simulink model "t04_combine_gaits_sol"  (R2024b)
settings: Solver=ode23t  StartTime=0.0  StopTime=4  RelTol=1e-3  AbsTol=1e-3  EnableMultiTasking=on
model workspace (MAT data in the model file):
  A = 0.4
  Critical_Velocity = 0.01
  Damping_Factor = 1000
  Dynamic_Friction = 0.5
  Heigth_brick : Simulink.Parameter (value not decoded)
  Heigth_ramp : Simulink.Parameter (value not decoded)
  Length_brick : Simulink.Parameter (value not decoded)
  Length_ramp : Simulink.Parameter (value not decoded)
  Length_torso : Simulink.Parameter (value not decoded)
  Lower_limbs : Simulink.Parameter (value not decoded)
  Static_Friction = 0.7
  Stiffnesscoefficient = 10000
  Transition_Region_Width = 0.02
  Upper_limbs : Simulink.Parameter (value not decoded)
  Width_brick : Simulink.Parameter (value not decoded)
  Width_ramp : Simulink.Parameter (value not decoded)
  Width_torso : Simulink.Parameter (value not decoded)
  f = 1.5
  max_Joint_change = 100
  r_foot : Simulink.Parameter (value not decoded)
  sampleTime : Simulink.Parameter (value not decoded)
  t_leg : Simulink.Parameter (value not decoded)
  theta : Simulink.Parameter (value not decoded)
  transferFunVal : Simulink.Parameter (value not decoded)
symbols that are objects in the model workspace (value not decoded): Length_torso, Lower_limbs, t_leg, Upper_limbs, Width_torso
undefined symbols (not defined in the file): X, Y, Z
libraries: sm_lib x78, nesl_utility x13
(part 3 of 4)

== system t04_combine_gaits_sol/Front left leg/Upper Limb ==
  BaseUpperLimb : sm_lib/Body Elements/Brick Solid  BrickDimensions=[t_leg t_leg L]  BrickDimensionsUnits=m  ExportEntireGeometry=off  InertiaType=CalculateFromGeometry  BasedOnType=Density  Density=1000  DensityUnits=kg/m^3  Mass=1  MassUnits=kg  CenterOfMass=[0 0 0]  CenterOfMassUnits=m  MomentsOfInertia=[1 1 1]  MomentsOfInertiaUnits=kg*m^2  ProductsOfInertia=[0 0 0]  ProductsOfInertiaUnits=kg*m^2  GraphicType=FromGeometry  MarkerShape=Sphere  MarkerSize=10  GraphicVisPropType=SimpleVisualProperties  GraphicDiffuseColor=[0.3922 0.8314 0.07451]  GraphicOpacity=1  GraphicSpecularColor=[0.5 0.5 0.5 1.0]  GraphicAmbientColor=[0.15 0.15 0.15 1.0]  GraphicEmissiveColor=[0.0 0.0 0.0 1.0]  GraphicShininess=75  DoExposeReferenceFrame=off  SerializedFrames=<Frames><Frame><Id>Frame1</Id><Value><Name>B</Name><Origin><Source>GeometricFeature</Source><FeatureName>+z surface</FeatureName></Origin><PrimaryAxis><DefinedDirection>+Z</DefinedDirection><Source>ReferenceFrame</Source><SourceDirection>+Z</SourceDirection><FeatureName></FeatureName></PrimaryAxis><SecondaryAxis><DefinedDirection>+X</DefinedDirection><Source>ReferenceFrame</Source><SourceDirection>+X</SourceDirection><FeatureName></FeatureName></SecondaryAxis></Value></Frame><Frame><Id>Frame2</Id><Value><Name>F</Name><Origin><Source>GeometricFeature</Source><FeatureName>-z surface</FeatureName></Origin><PrimaryAxis><DefinedDirection>+Z</DefinedDirection><Source>ReferenceFrame</Source><SourceDirection>+Z</SourceDirection><FeatureName></FeatureName></PrimaryAxis><SecondaryAxis><DefinedDirection>+X</DefinedDirection><Source>ReferenceFrame</Source><SourceDirection>+X</SourceDirection><FeatureName></FeatureName></SecondaryAxis></Value></Frame></Frames>
  Transform Shoulder : sm_lib/Frames and Transforms/Rigid Transform  RotationMethod=StandardAxis  FollAlignAxisA=+X  BaseAlignAxisA=+Y  FollAlignAxisB=+Y  BaseAlignAxisB=+Z  RotationStandardAxis=+X  RotationAngle=-90  RotationAngleUnits=deg  RotationArbitraryAxis=[0 0 1]  RotationSequenceAxes=FollowerAxes  RotationSequence=XYX  RotationSequenceAngles=[0 0 0]  RotationSequenceAnglesUnits=deg  RotationMatrix=[1 0 0;0 1 0;0 0 1]  Quaternion=[1 0 0 0]  TranslationMethod=StandardAxis  TranslationCartesianOffset=[0 0 0]  TranslationCartesianOffsetUnits=m  TranslationStandardAxis=+Z  TranslationStandardOffset=0  TranslationStandardOffsetUnits=m  TranslationROffset=0  TranslationROffsetUnits=m  TranslationThetaOffset=0  TranslationThetaOffsetUnits=deg  TranslationZOffset=0  TranslationZOffsetUnits=m
  Transform Upper Knee : sm_lib/Frames and Transforms/Rigid Transform  RotationMethod=StandardAxis  FollAlignAxisA=+X  BaseAlignAxisA=+Y  FollAlignAxisB=+Y  BaseAlignAxisB=+Z  RotationStandardAxis=+X  RotationAngle=-90  RotationAngleUnits=deg  RotationArbitraryAxis=[0 0 1]  RotationSequenceAxes=FollowerAxes  RotationSequence=XYX  RotationSequenceAngles=[0 0 0]  RotationSequenceAnglesUnits=deg  RotationMatrix=[1 0 0;0 1 0;0 0 1]  Quaternion=[1 0 0 0]  TranslationMethod=StandardAxis  TranslationCartesianOffset=[0 0 0]  TranslationCartesianOffsetUnits=m  TranslationStandardAxis=+Z  TranslationStandardOffset=0  TranslationStandardOffsetUnits=m  TranslationROffset=0  TranslationROffsetUnits=m  TranslationThetaOffset=0  TranslationThetaOffsetUnits=deg  TranslationZOffset=0  TranslationZOffsetUnits=m
  U : PMIOPort  Side=Left
  L : PMIOPort  Port=2  Side=Right
  connections:
  L/RConn1 -- Transform Upper Knee/RConn1
  U/RConn1 -- Transform Shoulder/RConn1
  BaseUpperLimb/LConn1 -- Transform Shoulder/LConn1
  BaseUpperLimb/RConn1 -- Transform Upper Knee/LConn1

== system t04_combine_gaits_sol/Front right leg/Lower Limb ==
  BaseLowerLimb : sm_lib/Body Elements/Brick Solid  BrickDimensions=[t_leg t_leg L]  BrickDimensionsUnits=m  ExportEntireGeometry=off  InertiaType=CalculateFromGeometry  BasedOnType=Density  Density=1000  DensityUnits=kg/m^3  Mass=1  MassUnits=kg  CenterOfMass=[0 0 0]  CenterOfMassUnits=m  MomentsOfInertia=[1 1 1]  MomentsOfInertiaUnits=kg*m^2  ProductsOfInertia=[0 0 0]  ProductsOfInertiaUnits=kg*m^2  GraphicType=FromGeometry  MarkerShape=Sphere  MarkerSize=10  GraphicVisPropType=SimpleVisualProperties  GraphicDiffuseColor=[0.3922 0.8314 0.07451]  GraphicOpacity=1  GraphicSpecularColor=[0.5 0.5 0.5 1.0]  GraphicAmbientColor=[0.15 0.15 0.15 1.0]  GraphicEmissiveColor=[0.0 0.0 0.0 1.0]  GraphicShininess=75  DoExposeReferenceFrame=off  SerializedFrames=<Frames><Frame><Id>Frame1</Id><Value><Name>B</Name><Origin><Source>GeometricFeature</Source><FeatureName>+z surface</FeatureName></Origin><PrimaryAxis><DefinedDirection>+Z</DefinedDirection><Source>ReferenceFrame</Source><SourceDirection>+Z</SourceDirection><FeatureName></FeatureName></PrimaryAxis><SecondaryAxis><DefinedDirection>+X</DefinedDirection><Source>ReferenceFrame</Source><SourceDirection>+X</SourceDirection><FeatureName></FeatureName></SecondaryAxis></Value></Frame><Frame><Id>Frame2</Id><Value><Name>F</Name><Origin><Source>GeometricFeature</Source><FeatureName>-z surface</FeatureName></Origin><PrimaryAxis><DefinedDirection>+Z</DefinedDirection><Source>ReferenceFrame</Source><SourceDirection>+Z</SourceDirection><FeatureName></FeatureName></PrimaryAxis><SecondaryAxis><DefinedDirection>+X</DefinedDirection><Source>ReferenceFrame</Source><SourceDirection>+X</SourceDirection><FeatureName></FeatureName></SecondaryAxis></Value></Frame></Frames>
  Transform Shoulder : sm_lib/Frames and Transforms/Rigid Transform  RotationMethod=StandardAxis  FollAlignAxisA=+X  BaseAlignAxisA=+Y  FollAlignAxisB=+Y  BaseAlignAxisB=+Z  RotationStandardAxis=+X  RotationAngle=-90  RotationAngleUnits=deg  RotationArbitraryAxis=[0 0 1]  RotationSequenceAxes=FollowerAxes  RotationSequence=XYX  RotationSequenceAngles=[0 0 0]  RotationSequenceAnglesUnits=deg  RotationMatrix=[1 0 0;0 1 0;0 0 1]  Quaternion=[1 0 0 0]  TranslationMethod=StandardAxis  TranslationCartesianOffset=[0 0 0]  TranslationCartesianOffsetUnits=m  TranslationStandardAxis=+Z  TranslationStandardOffset=0  TranslationStandardOffsetUnits=m  TranslationROffset=0  TranslationROffsetUnits=m  TranslationThetaOffset=0  TranslationThetaOffsetUnits=deg  TranslationZOffset=0  TranslationZOffsetUnits=m
  Transform Upper Knee : sm_lib/Frames and Transforms/Rigid Transform  RotationMethod=StandardAxis  FollAlignAxisA=+X  BaseAlignAxisA=+Y  FollAlignAxisB=+Y  BaseAlignAxisB=+Z  RotationStandardAxis=+X  RotationAngle=-90  RotationAngleUnits=deg  RotationArbitraryAxis=[0 0 1]  RotationSequenceAxes=FollowerAxes  RotationSequence=XYX  RotationSequenceAngles=[0 0 0]  RotationSequenceAnglesUnits=deg  RotationMatrix=[1 0 0;0 1 0;0 0 1]  Quaternion=[1 0 0 0]  TranslationMethod=StandardAxis  TranslationCartesianOffset=[0 0 0]  TranslationCartesianOffsetUnits=m  TranslationStandardAxis=+Z  TranslationStandardOffset=0  TranslationStandardOffsetUnits=m  TranslationROffset=0  TranslationROffsetUnits=m  TranslationThetaOffset=0  TranslationThetaOffsetUnits=deg  TranslationZOffset=0  TranslationZOffsetUnits=m
  U : PMIOPort  Side=Left
  L : PMIOPort  Port=2  Side=Right
  connections:
  BaseLowerLimb/LConn1 -- Transform Shoulder/LConn1
  Transform Shoulder/RConn1 -- U/RConn1
  L/RConn1 -- Transform Upper Knee/RConn1
  BaseLowerLimb/RConn1 -- Transform Upper Knee/LConn1

== system t04_combine_gaits_sol/Front right leg/Upper Limb ==
  BaseUpperLimb : sm_lib/Body Elements/Brick Solid  BrickDimensions=[t_leg t_leg L]  BrickDimensionsUnits=m  ExportEntireGeometry=off  InertiaType=CalculateFromGeometry  BasedOnType=Density  Density=1000  DensityUnits=kg/m^3  Mass=1  MassUnits=kg  CenterOfMass=[0 0 0]  CenterOfMassUnits=m  MomentsOfInertia=[1 1 1]  MomentsOfInertiaUnits=kg*m^2  ProductsOfInertia=[0 0 0]  ProductsOfInertiaUnits=kg*m^2  GraphicType=FromGeometry  MarkerShape=Sphere  MarkerSize=10  GraphicVisPropType=SimpleVisualProperties  GraphicDiffuseColor=[0.3922 0.8314 0.07451]  GraphicOpacity=1  GraphicSpecularColor=[0.5 0.5 0.5 1.0]  GraphicAmbientColor=[0.15 0.15 0.15 1.0]  GraphicEmissiveColor=[0.0 0.0 0.0 1.0]  GraphicShininess=75  DoExposeReferenceFrame=off  SerializedFrames=<Frames><Frame><Id>Frame1</Id><Value><Name>B</Name><Origin><Source>GeometricFeature</Source><FeatureName>+z surface</FeatureName></Origin><PrimaryAxis><DefinedDirection>+Z</DefinedDirection><Source>ReferenceFrame</Source><SourceDirection>+Z</SourceDirection><FeatureName></FeatureName></PrimaryAxis><SecondaryAxis><DefinedDirection>+X</DefinedDirection><Source>ReferenceFrame</Source><SourceDirection>+X</SourceDirection><FeatureName></FeatureName></SecondaryAxis></Value></Frame><Frame><Id>Frame2</Id><Value><Name>F</Name><Origin><Source>GeometricFeature</Source><FeatureName>-z surface</FeatureName></Origin><PrimaryAxis><DefinedDirection>+Z</DefinedDirection><Source>ReferenceFrame</Source><SourceDirection>+Z</SourceDirection><FeatureName></FeatureName></PrimaryAxis><SecondaryAxis><DefinedDirection>+X</DefinedDirection><Source>ReferenceFrame</Source><SourceDirection>+X</SourceDirection><FeatureName></FeatureName></SecondaryAxis></Value></Frame></Frames>
  Transform Shoulder : sm_lib/Frames and Transforms/Rigid Transform  RotationMethod=StandardAxis  FollAlignAxisA=+X  BaseAlignAxisA=+Y  FollAlignAxisB=+Y  BaseAlignAxisB=+Z  RotationStandardAxis=+X  RotationAngle=-90  RotationAngleUnits=deg  RotationArbitraryAxis=[0 0 1]  RotationSequenceAxes=FollowerAxes  RotationSequence=XYX  RotationSequenceAngles=[0 0 0]  RotationSequenceAnglesUnits=deg  RotationMatrix=[1 0 0;0 1 0;0 0 1]  Quaternion=[1 0 0 0]  TranslationMethod=StandardAxis  TranslationCartesianOffset=[0 0 0]  TranslationCartesianOffsetUnits=m  TranslationStandardAxis=+Z  TranslationStandardOffset=0  TranslationStandardOffsetUnits=m  TranslationROffset=0  TranslationROffsetUnits=m  TranslationThetaOffset=0  TranslationThetaOffsetUnits=deg  TranslationZOffset=0  TranslationZOffsetUnits=m
  Transform Upper Knee : sm_lib/Frames and Transforms/Rigid Transform  RotationMethod=StandardAxis  FollAlignAxisA=+X  BaseAlignAxisA=+Y  FollAlignAxisB=+Y  BaseAlignAxisB=+Z  RotationStandardAxis=+X  RotationAngle=-90  RotationAngleUnits=deg  RotationArbitraryAxis=[0 0 1]  RotationSequenceAxes=FollowerAxes  RotationSequence=XYX  RotationSequenceAngles=[0 0 0]  RotationSequenceAnglesUnits=deg  RotationMatrix=[1 0 0;0 1 0;0 0 1]  Quaternion=[1 0 0 0]  TranslationMethod=StandardAxis  TranslationCartesianOffset=[0 0 0]  TranslationCartesianOffsetUnits=m  TranslationStandardAxis=+Z  TranslationStandardOffset=0  TranslationStandardOffsetUnits=m  TranslationROffset=0  TranslationROffsetUnits=m  TranslationThetaOffset=0  TranslationThetaOffsetUnits=deg  TranslationZOffset=0  TranslationZOffsetUnits=m
  U : PMIOPort  Side=Left
  L : PMIOPort  Port=2  Side=Right
  connections:
  L/RConn1 -- Transform Upper Knee/RConn1
  U/RConn1 -- Transform Shoulder/RConn1
  BaseUpperLimb/LConn1 -- Transform Shoulder/LConn1
  BaseUpperLimb/RConn1 -- Transform Upper Knee/LConn1

== system t04_combine_gaits_sol/Rear left leg/Lower Limb ==
  BaseLowerLimb : sm_lib/Body Elements/Brick Solid  BrickDimensions=[t_leg t_leg L]  BrickDimensionsUnits=m  ExportEntireGeometry=off  InertiaType=CalculateFromGeometry  BasedOnType=Density  Density=1000  DensityUnits=kg/m^3  Mass=1  MassUnits=kg  CenterOfMass=[0 0 0]  CenterOfMassUnits=m  MomentsOfInertia=[1 1 1]  MomentsOfInertiaUnits=kg*m^2  ProductsOfInertia=[0 0 0]  ProductsOfInertiaUnits=kg*m^2  GraphicType=FromGeometry  MarkerShape=Sphere  MarkerSize=10  GraphicVisPropType=SimpleVisualProperties  GraphicDiffuseColor=[0.3922 0.8314 0.07451]  GraphicOpacity=1  GraphicSpecularColor=[0.5 0.5 0.5 1.0]  GraphicAmbientColor=[0.15 0.15 0.15 1.0]  GraphicEmissiveColor=[0.0 0.0 0.0 1.0]  GraphicShininess=75  DoExposeReferenceFrame=off  SerializedFrames=<Frames><Frame><Id>Frame1</Id><Value><Name>B</Name><Origin><Source>GeometricFeature</Source><FeatureName>+z surface</FeatureName></Origin><PrimaryAxis><DefinedDirection>+Z</DefinedDirection><Source>ReferenceFrame</Source><SourceDirection>+Z</SourceDirection><FeatureName></FeatureName></PrimaryAxis><SecondaryAxis><DefinedDirection>+X</DefinedDirection><Source>ReferenceFrame</Source><SourceDirection>+X</SourceDirection><FeatureName></FeatureName></SecondaryAxis></Value></Frame><Frame><Id>Frame2</Id><Value><Name>F</Name><Origin><Source>GeometricFeature</Source><FeatureName>-z surface</FeatureName></Origin><PrimaryAxis><DefinedDirection>+Z</DefinedDirection><Source>ReferenceFrame</Source><SourceDirection>+Z</SourceDirection><FeatureName></FeatureName></PrimaryAxis><SecondaryAxis><DefinedDirection>+X</DefinedDirection><Source>ReferenceFrame</Source><SourceDirection>+X</SourceDirection><FeatureName></FeatureName></SecondaryAxis></Value></Frame></Frames>
  Transform Shoulder : sm_lib/Frames and Transforms/Rigid Transform  RotationMethod=StandardAxis  FollAlignAxisA=+X  BaseAlignAxisA=+Y  FollAlignAxisB=+Y  BaseAlignAxisB=+Z  RotationStandardAxis=+X  RotationAngle=-90  RotationAngleUnits=deg  RotationArbitraryAxis=[0 0 1]  RotationSequenceAxes=FollowerAxes  RotationSequence=XYX  RotationSequenceAngles=[0 0 0]  RotationSequenceAnglesUnits=deg  RotationMatrix=[1 0 0;0 1 0;0 0 1]  Quaternion=[1 0 0 0]  TranslationMethod=StandardAxis  TranslationCartesianOffset=[0 0 0]  TranslationCartesianOffsetUnits=m  TranslationStandardAxis=+Z  TranslationStandardOffset=0  TranslationStandardOffsetUnits=m  TranslationROffset=0  TranslationROffsetUnits=m  TranslationThetaOffset=0  TranslationThetaOffsetUnits=deg  TranslationZOffset=0  TranslationZOffsetUnits=m
  Transform Upper Knee : sm_lib/Frames and Transforms/Rigid Transform  RotationMethod=StandardAxis  FollAlignAxisA=+X  BaseAlignAxisA=+Y  FollAlignAxisB=+Y  BaseAlignAxisB=+Z  RotationStandardAxis=+X  RotationAngle=-90  RotationAngleUnits=deg  RotationArbitraryAxis=[0 0 1]  RotationSequenceAxes=FollowerAxes  RotationSequence=XYX  RotationSequenceAngles=[0 0 0]  RotationSequenceAnglesUnits=deg  RotationMatrix=[1 0 0;0 1 0;0 0 1]  Quaternion=[1 0 0 0]  TranslationMethod=StandardAxis  TranslationCartesianOffset=[0 0 0]  TranslationCartesianOffsetUnits=m  TranslationStandardAxis=+Z  TranslationStandardOffset=0  TranslationStandardOffsetUnits=m  TranslationROffset=0  TranslationROffsetUnits=m  TranslationThetaOffset=0  TranslationThetaOffsetUnits=deg  TranslationZOffset=0  TranslationZOffsetUnits=m
  U : PMIOPort  Side=Left
  L : PMIOPort  Port=2  Side=Right
  connections:
  BaseLowerLimb/LConn1 -- Transform Shoulder/LConn1
  Transform Shoulder/RConn1 -- U/RConn1
  L/RConn1 -- Transform Upper Knee/RConn1
  BaseLowerLimb/RConn1 -- Transform Upper Knee/LConn1

== system t04_combine_gaits_sol/Rear left leg/Upper Limb ==
  BaseUpperLimb : sm_lib/Body Elements/Brick Solid  BrickDimensions=[t_leg t_leg L]  BrickDimensionsUnits=m  ExportEntireGeometry=off  InertiaType=CalculateFromGeometry  BasedOnType=Density  Density=1000  DensityUnits=kg/m^3  Mass=1  MassUnits=kg  CenterOfMass=[0 0 0]  CenterOfMassUnits=m  MomentsOfInertia=[1 1 1]  MomentsOfInertiaUnits=kg*m^2  ProductsOfInertia=[0 0 0]  ProductsOfInertiaUnits=kg*m^2  GraphicType=FromGeometry  MarkerShape=Sphere  MarkerSize=10  GraphicVisPropType=SimpleVisualProperties  GraphicDiffuseColor=[0.3922 0.8314 0.07451]  GraphicOpacity=1  GraphicSpecularColor=[0.5 0.5 0.5 1.0]  GraphicAmbientColor=[0.15 0.15 0.15 1.0]  GraphicEmissiveColor=[0.0 0.0 0.0 1.0]  GraphicShininess=75  DoExposeReferenceFrame=off  SerializedFrames=<Frames><Frame><Id>Frame1</Id><Value><Name>B</Name><Origin><Source>GeometricFeature</Source><FeatureName>+z surface</FeatureName></Origin><PrimaryAxis><DefinedDirection>+Z</DefinedDirection><Source>ReferenceFrame</Source><SourceDirection>+Z</SourceDirection><FeatureName></FeatureName></PrimaryAxis><SecondaryAxis><DefinedDirection>+X</DefinedDirection><Source>ReferenceFrame</Source><SourceDirection>+X</SourceDirection><FeatureName></FeatureName></SecondaryAxis></Value></Frame><Frame><Id>Frame2</Id><Value><Name>F</Name><Origin><Source>GeometricFeature</Source><FeatureName>-z surface</FeatureName></Origin><PrimaryAxis><DefinedDirection>+Z</DefinedDirection><Source>ReferenceFrame</Source><SourceDirection>+Z</SourceDirection><FeatureName></FeatureName></PrimaryAxis><SecondaryAxis><DefinedDirection>+X</DefinedDirection><Source>ReferenceFrame</Source><SourceDirection>+X</SourceDirection><FeatureName></FeatureName></SecondaryAxis></Value></Frame></Frames>
  Transform Shoulder : sm_lib/Frames and Transforms/Rigid Transform  RotationMethod=StandardAxis  FollAlignAxisA=+X  BaseAlignAxisA=+Y  FollAlignAxisB=+Y  BaseAlignAxisB=+Z  RotationStandardAxis=+X  RotationAngle=-90  RotationAngleUnits=deg  RotationArbitraryAxis=[0 0 1]  RotationSequenceAxes=FollowerAxes  RotationSequence=XYX  RotationSequenceAngles=[0 0 0]  RotationSequenceAnglesUnits=deg  RotationMatrix=[1 0 0;0 1 0;0 0 1]  Quaternion=[1 0 0 0]  TranslationMethod=StandardAxis  TranslationCartesianOffset=[0 0 0]  TranslationCartesianOffsetUnits=m  TranslationStandardAxis=+Z  TranslationStandardOffset=0  TranslationStandardOffsetUnits=m  TranslationROffset=0  TranslationROffsetUnits=m  TranslationThetaOffset=0  TranslationThetaOffsetUnits=deg  TranslationZOffset=0  TranslationZOffsetUnits=m
  Transform Upper Knee : sm_lib/Frames and Transforms/Rigid Transform  RotationMethod=StandardAxis  FollAlignAxisA=+X  BaseAlignAxisA=+Y  FollAlignAxisB=+Y  BaseAlignAxisB=+Z  RotationStandardAxis=+X  RotationAngle=-90  RotationAngleUnits=deg  RotationArbitraryAxis=[0 0 1]  RotationSequenceAxes=FollowerAxes  RotationSequence=XYX  RotationSequenceAngles=[0 0 0]  RotationSequenceAnglesUnits=deg  RotationMatrix=[1 0 0;0 1 0;0 0 1]  Quaternion=[1 0 0 0]  TranslationMethod=StandardAxis  TranslationCartesianOffset=[0 0 0]  TranslationCartesianOffsetUnits=m  TranslationStandardAxis=+Z  TranslationStandardOffset=0  TranslationStandardOffsetUnits=m  TranslationROffset=0  TranslationROffsetUnits=m  TranslationThetaOffset=0  TranslationThetaOffsetUnits=deg  TranslationZOffset=0  TranslationZOffsetUnits=m
  U : PMIOPort  Side=Left
  L : PMIOPort  Port=2  Side=Right
  connections:
  L/RConn1 -- Transform Upper Knee/RConn1
  U/RConn1 -- Transform Shoulder/RConn1
  BaseUpperLimb/LConn1 -- Transform Shoulder/LConn1
  BaseUpperLimb/RConn1 -- Transform Upper Knee/LConn1

== system t04_combine_gaits_sol/Rear right leg/Lower Limb ==
  BaseLowerLimb : sm_lib/Body Elements/Brick Solid  BrickDimensions=[t_leg t_leg L]  BrickDimensionsUnits=m  ExportEntireGeometry=off  InertiaType=CalculateFromGeometry  BasedOnType=Density  Density=1000  DensityUnits=kg/m^3  Mass=1  MassUnits=kg  CenterOfMass=[0 0 0]  CenterOfMassUnits=m  MomentsOfInertia=[1 1 1]  MomentsOfInertiaUnits=kg*m^2  ProductsOfInertia=[0 0 0]  ProductsOfInertiaUnits=kg*m^2  GraphicType=FromGeometry  MarkerShape=Sphere  MarkerSize=10  GraphicVisPropType=SimpleVisualProperties  GraphicDiffuseColor=[0.3922 0.8314 0.07451]  GraphicOpacity=1  GraphicSpecularColor=[0.5 0.5 0.5 1.0]  GraphicAmbientColor=[0.15 0.15 0.15 1.0]  GraphicEmissiveColor=[0.0 0.0 0.0 1.0]  GraphicShininess=75  DoExposeReferenceFrame=off  SerializedFrames=<Frames><Frame><Id>Frame1</Id><Value><Name>B</Name><Origin><Source>GeometricFeature</Source><FeatureName>+z surface</FeatureName></Origin><PrimaryAxis><DefinedDirection>+Z</DefinedDirection><Source>ReferenceFrame</Source><SourceDirection>+Z</SourceDirection><FeatureName></FeatureName></PrimaryAxis><SecondaryAxis><DefinedDirection>+X</DefinedDirection><Source>ReferenceFrame</Source><SourceDirection>+X</SourceDirection><FeatureName></FeatureName></SecondaryAxis></Value></Frame><Frame><Id>Frame2</Id><Value><Name>F</Name><Origin><Source>GeometricFeature</Source><FeatureName>-z surface</FeatureName></Origin><PrimaryAxis><DefinedDirection>+Z</DefinedDirection><Source>ReferenceFrame</Source><SourceDirection>+Z</SourceDirection><FeatureName></FeatureName></PrimaryAxis><SecondaryAxis><DefinedDirection>+X</DefinedDirection><Source>ReferenceFrame</Source><SourceDirection>+X</SourceDirection><FeatureName></FeatureName></SecondaryAxis></Value></Frame></Frames>
  Transform Shoulder : sm_lib/Frames and Transforms/Rigid Transform  RotationMethod=StandardAxis  FollAlignAxisA=+X  BaseAlignAxisA=+Y  FollAlignAxisB=+Y  BaseAlignAxisB=+Z  RotationStandardAxis=+X  RotationAngle=-90  RotationAngleUnits=deg  RotationArbitraryAxis=[0 0 1]  RotationSequenceAxes=FollowerAxes  RotationSequence=XYX  RotationSequenceAngles=[0 0 0]  RotationSequenceAnglesUnits=deg  RotationMatrix=[1 0 0;0 1 0;0 0 1]  Quaternion=[1 0 0 0]  TranslationMethod=StandardAxis  TranslationCartesianOffset=[0 0 0]  TranslationCartesianOffsetUnits=m  TranslationStandardAxis=+Z  TranslationStandardOffset=0  TranslationStandardOffsetUnits=m  TranslationROffset=0  TranslationROffsetUnits=m  TranslationThetaOffset=0  TranslationThetaOffsetUnits=deg  TranslationZOffset=0  TranslationZOffsetUnits=m
  Transform Upper Knee : sm_lib/Frames and Transforms/Rigid Transform  RotationMethod=StandardAxis  FollAlignAxisA=+X  BaseAlignAxisA=+Y  FollAlignAxisB=+Y  BaseAlignAxisB=+Z  RotationStandardAxis=+X  RotationAngle=-90  RotationAngleUnits=deg  RotationArbitraryAxis=[0 0 1]  RotationSequenceAxes=FollowerAxes  RotationSequence=XYX  RotationSequenceAngles=[0 0 0]  RotationSequenceAnglesUnits=deg  RotationMatrix=[1 0 0;0 1 0;0 0 1]  Quaternion=[1 0 0 0]  TranslationMethod=StandardAxis  TranslationCartesianOffset=[0 0 0]  TranslationCartesianOffsetUnits=m  TranslationStandardAxis=+Z  TranslationStandardOffset=0  TranslationStandardOffsetUnits=m  TranslationROffset=0  TranslationROffsetUnits=m  TranslationThetaOffset=0  TranslationThetaOffsetUnits=deg  TranslationZOffset=0  TranslationZOffsetUnits=m
  U : PMIOPort  Side=Left
  L : PMIOPort  Port=2  Side=Right
  connections:
  BaseLowerLimb/LConn1 -- Transform Shoulder/LConn1
  Transform Shoulder/RConn1 -- U/RConn1
  L/RConn1 -- Transform Upper Knee/RConn1
  BaseLowerLimb/RConn1 -- Transform Upper Knee/LConn1

== system t04_combine_gaits_sol/Rear right leg/Upper Limb ==
  BaseUpperLimb : sm_lib/Body Elements/Brick Solid  BrickDimensions=[t_leg t_leg L]  BrickDimensionsUnits=m  ExportEntireGeometry=off  InertiaType=CalculateFromGeometry  BasedOnType=Density  Density=1000  DensityUnits=kg/m^3  Mass=1  MassUnits=kg  CenterOfMass=[0 0 0]  CenterOfMassUnits=m  MomentsOfInertia=[1 1 1]  MomentsOfInertiaUnits=kg*m^2  ProductsOfInertia=[0 0 0]  ProductsOfInertiaUnits=kg*m^2  GraphicType=FromGeometry  MarkerShape=Sphere  MarkerSize=10  GraphicVisPropType=SimpleVisualProperties  GraphicDiffuseColor=[0.3922 0.8314 0.07451]  GraphicOpacity=1  GraphicSpecularColor=[0.5 0.5 0.5 1.0]  GraphicAmbientColor=[0.15 0.15 0.15 1.0]  GraphicEmissiveColor=[0.0 0.0 0.0 1.0]  GraphicShininess=75  DoExposeReferenceFrame=off  SerializedFrames=<Frames><Frame><Id>Frame1</Id><Value><Name>B</Name><Origin><Source>GeometricFeature</Source><FeatureName>+z surface</FeatureName></Origin><PrimaryAxis><DefinedDirection>+Z</DefinedDirection><Source>ReferenceFrame</Source><SourceDirection>+Z</SourceDirection><FeatureName></FeatureName></PrimaryAxis><SecondaryAxis><DefinedDirection>+X</DefinedDirection><Source>ReferenceFrame</Source><SourceDirection>+X</SourceDirection><FeatureName></FeatureName></SecondaryAxis></Value></Frame><Frame><Id>Frame2</Id><Value><Name>F</Name><Origin><Source>GeometricFeature</Source><FeatureName>-z surface</FeatureName></Origin><PrimaryAxis><DefinedDirection>+Z</DefinedDirection><Source>ReferenceFrame</Source><SourceDirection>+Z</SourceDirection><FeatureName></FeatureName></PrimaryAxis><SecondaryAxis><DefinedDirection>+X</DefinedDirection><Source>ReferenceFrame</Source><SourceDirection>+X</SourceDirection><FeatureName></FeatureName></SecondaryAxis></Value></Frame></Frames>
  Transform Shoulder : sm_lib/Frames and Transforms/Rigid Transform  RotationMethod=StandardAxis  FollAlignAxisA=+X  BaseAlignAxisA=+Y  FollAlignAxisB=+Y  BaseAlignAxisB=+Z  RotationStandardAxis=+X  RotationAngle=-90  RotationAngleUnits=deg  RotationArbitraryAxis=[0 0 1]  RotationSequenceAxes=FollowerAxes  RotationSequence=XYX  RotationSequenceAngles=[0 0 0]  RotationSequenceAnglesUnits=deg  RotationMatrix=[1 0 0;0 1 0;0 0 1]  Quaternion=[1 0 0 0]  TranslationMethod=StandardAxis  TranslationCartesianOffset=[0 0 0]  TranslationCartesianOffsetUnits=m  TranslationStandardAxis=+Z  TranslationStandardOffset=0  TranslationStandardOffsetUnits=m  TranslationROffset=0  TranslationROffsetUnits=m  TranslationThetaOffset=0  TranslationThetaOffsetUnits=deg  TranslationZOffset=0  TranslationZOffsetUnits=m
  Transform Upper Knee : sm_lib/Frames and Transforms/Rigid Transform  RotationMethod=StandardAxis  FollAlignAxisA=+X  BaseAlignAxisA=+Y  FollAlignAxisB=+Y  BaseAlignAxisB=+Z  RotationStandardAxis=+X  RotationAngle=-90  RotationAngleUnits=deg  RotationArbitraryAxis=[0 0 1]  RotationSequenceAxes=FollowerAxes  RotationSequence=XYX  RotationSequenceAngles=[0 0 0]  RotationSequenceAnglesUnits=deg  RotationMatrix=[1 0 0;0 1 0;0 0 1]  Quaternion=[1 0 0 0]  TranslationMethod=StandardAxis  TranslationCartesianOffset=[0 0 0]  TranslationCartesianOffsetUnits=m  TranslationStandardAxis=+Z  TranslationStandardOffset=0  TranslationStandardOffsetUnits=m  TranslationROffset=0  TranslationROffsetUnits=m  TranslationThetaOffset=0  TranslationThetaOffsetUnits=deg  TranslationZOffset=0  TranslationZOffsetUnits=m
  U : PMIOPort  Side=Left
  L : PMIOPort  Port=2  Side=Right
  connections:
  L/RConn1 -- Transform Upper Knee/RConn1
  U/RConn1 -- Transform Shoulder/RConn1
  BaseUpperLimb/LConn1 -- Transform Shoulder/LConn1
  BaseUpperLimb/RConn1 -- Transform Upper Knee/LConn1

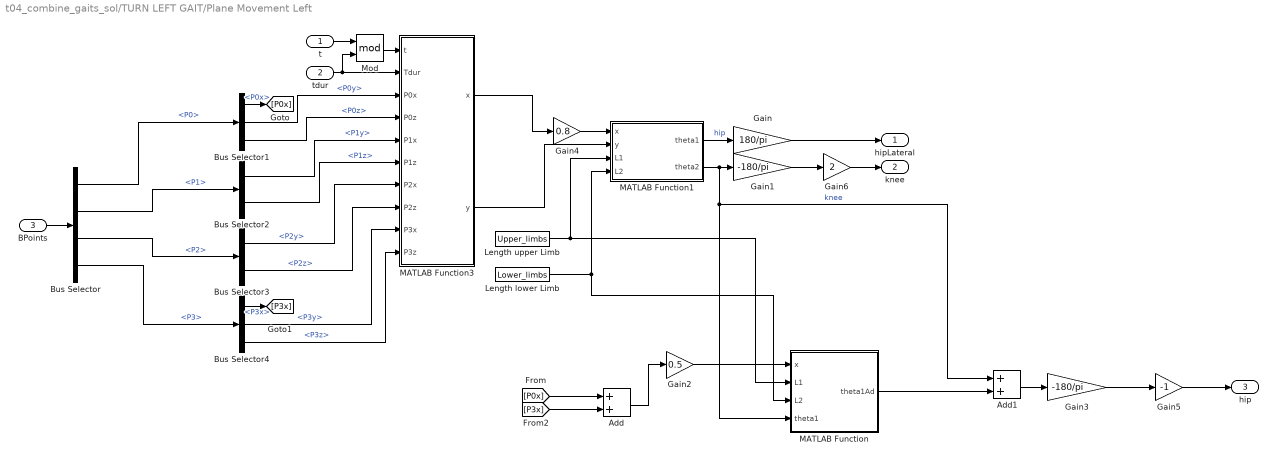
== system t04_combine_gaits_sol/TURN LEFT GAIT/Plane Movement Left ==
  t : Inport
  tdur : Inport  Port=2
  BPoints : Inport  Port=3
  Add : Sum
  Add1 : Sum
  Bus Selector : BusSelector  OutputSignals=P0,P1,P2,P3
  Bus Selector1 : BusSelector  OutputSignals=P0x,P0y,P0z
  Bus Selector2 : BusSelector  OutputSignals=P1y,P1z
  Bus Selector3 : BusSelector  OutputSignals=P2y,P2z
  Bus Selector4 : BusSelector  OutputSignals=P3x,P3y,P3z
  Gain : Gain  Gain=180/pi
  Gain1 : Gain  Gain=-180/pi
  Gain2 : Gain  Gain=0.5
  Gain3 : Gain  Gain=-180/pi
  Gain4 : Gain  Gain=0.8
  Gain5 : Gain  Gain=-1
  Gain6 : Gain  Gain=2
  Length lower Limb : Constant  Value=Lower_limbs
  Length upper Limb : Constant  Value=Upper_limbs
  MATLAB Function : MATLAB Function  TreatAsAtomicUnit=on
  MATLAB Function1 : MATLAB Function  TreatAsAtomicUnit=on
  MATLAB Function3 : MATLAB Function  TreatAsAtomicUnit=on
  Mod : Math  Operator=mod
  hipLateral : Outport
  knee : Outport  Port=2
  hip : Outport  Port=3
  wires:
  Gain4/1 -> MATLAB Function1/1(x)
  Gain3/1 -> Gain5/1
  Add1/1 -> Gain3/1
  MATLAB Function/1(theta1Ad) -> Add1/2
  Bus Selector4/1 -> [P3x]  "<P3x>"
  Gain2/1 -> MATLAB Function/1(x)
  [P0x] -> Add/1
  [P3x] -> Add/2
  Add/1 -> Gain2/1
  Bus Selector1/1 -> [P0x]  "<P0x>"
  MATLAB Function3/2(y) -> MATLAB Function1/2(y)
  MATLAB Function3/1(x) -> Gain4/1
  MATLAB Function1/2(theta2) -> Gain1/1, MATLAB Function/4(theta1), Add1/1  "knee"
  tdur/1 -> Mod/2, MATLAB Function3/2(Tdur)
  MATLAB Function1/1(theta1) -> Gain/1  "hip"
  t/1 -> Mod/1
  Length upper Limb/1 -> MATLAB Function/2(L1), MATLAB Function1/3(L1)
  Length lower Limb/1 -> MATLAB Function/3(L2), MATLAB Function1/4(L2)
  Gain1/1 -> Gain6/1
  Gain/1 -> hipLateral/1
  Bus Selector/3 -> Bus Selector3/1  "<P2>"
  Bus Selector3/2 -> MATLAB Function3/8(P2z)  "<P2z>"
  Bus Selector2/1 -> MATLAB Function3/5(P1x)  "<P1y>"
  Bus Selector3/1 -> MATLAB Function3/7(P2x)  "<P2y>"
  Bus Selector4/2 -> MATLAB Function3/9(P3x)  "<P3y>"
  Bus Selector1/3 -> MATLAB Function3/4(P0z)  "<P0z>"
  Bus Selector/4 -> Bus Selector4/1  "<P3>"
  Bus Selector4/3 -> MATLAB Function3/10(P3z)  "<P3z>"
  Bus Selector/2 -> Bus Selector2/1  "<P1>"
  BPoints/1 -> Bus Selector/1
  Bus Selector1/2 -> MATLAB Function3/3(P0x)  "<P0y>"
  Bus Selector/1 -> Bus Selector1/1  "<P0>"
  Bus Selector2/2 -> MATLAB Function3/6(P1z)  "<P1z>"
  Mod/1 -> MATLAB Function3/1(t)
  Gain5/1 -> hip/1
  Gain6/1 -> knee/1

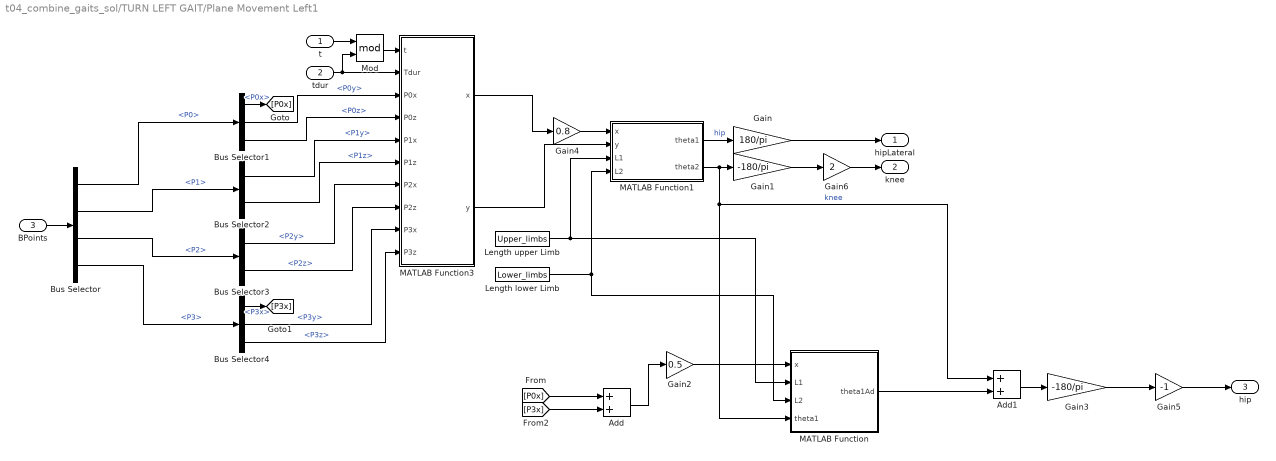
== system t04_combine_gaits_sol/TURN LEFT GAIT/Plane Movement Left1 ==
  t : Inport
  tdur : Inport  Port=2
  BPoints : Inport  Port=3
  Add : Sum
  Add1 : Sum
  Bus Selector : BusSelector  OutputSignals=P0,P1,P2,P3
  Bus Selector1 : BusSelector  OutputSignals=P0x,P0y,P0z
  Bus Selector2 : BusSelector  OutputSignals=P1y,P1z
  Bus Selector3 : BusSelector  OutputSignals=P2y,P2z
  Bus Selector4 : BusSelector  OutputSignals=P3x,P3y,P3z
  Gain : Gain  Gain=180/pi
  Gain1 : Gain  Gain=-180/pi
  Gain2 : Gain  Gain=0.5
  Gain3 : Gain  Gain=-180/pi
  Gain4 : Gain  Gain=0.8
  Gain5 : Gain  Gain=-1
  Gain6 : Gain  Gain=2
  Length lower Limb : Constant  Value=Lower_limbs
  Length upper Limb : Constant  Value=Upper_limbs
  MATLAB Function : MATLAB Function  TreatAsAtomicUnit=on
  MATLAB Function1 : MATLAB Function  TreatAsAtomicUnit=on
  MATLAB Function3 : MATLAB Function  TreatAsAtomicUnit=on
  Mod : Math  Operator=mod
  hipLateral : Outport
  knee : Outport  Port=2
  hip : Outport  Port=3
  wires:
  Gain4/1 -> MATLAB Function1/1(x)
  Gain3/1 -> Gain5/1
  Add1/1 -> Gain3/1
  MATLAB Function/1(theta1Ad) -> Add1/2
  Bus Selector4/1 -> [P3x]  "<P3x>"
  Gain2/1 -> MATLAB Function/1(x)
  [P0x] -> Add/1
  [P3x] -> Add/2
  Add/1 -> Gain2/1
  Bus Selector1/1 -> [P0x]  "<P0x>"
  MATLAB Function3/2(y) -> MATLAB Function1/2(y)
  MATLAB Function3/1(x) -> Gain4/1
  MATLAB Function1/2(theta2) -> Gain1/1, MATLAB Function/4(theta1), Add1/1  "knee"
  tdur/1 -> Mod/2, MATLAB Function3/2(Tdur)
  MATLAB Function1/1(theta1) -> Gain/1  "hip"
  t/1 -> Mod/1
  Length upper Limb/1 -> MATLAB Function/2(L1), MATLAB Function1/3(L1)
  Length lower Limb/1 -> MATLAB Function/3(L2), MATLAB Function1/4(L2)
  Gain1/1 -> Gain6/1
  Gain/1 -> hipLateral/1
  Bus Selector/3 -> Bus Selector3/1  "<P2>"
  Bus Selector3/2 -> MATLAB Function3/8(P2z)  "<P2z>"
  Bus Selector2/1 -> MATLAB Function3/5(P1x)  "<P1y>"
  Bus Selector3/1 -> MATLAB Function3/7(P2x)  "<P2y>"
  Bus Selector4/2 -> MATLAB Function3/9(P3x)  "<P3y>"
  Bus Selector1/3 -> MATLAB Function3/4(P0z)  "<P0z>"
  Bus Selector/4 -> Bus Selector4/1  "<P3>"
  Bus Selector4/3 -> MATLAB Function3/10(P3z)  "<P3z>"
  Bus Selector/2 -> Bus Selector2/1  "<P1>"
  BPoints/1 -> Bus Selector/1
  Bus Selector1/2 -> MATLAB Function3/3(P0x)  "<P0y>"
  Bus Selector/1 -> Bus Selector1/1  "<P0>"
  Bus Selector2/2 -> MATLAB Function3/6(P1z)  "<P1z>"
  Mod/1 -> MATLAB Function3/1(t)
  Gain5/1 -> hip/1
  Gain6/1 -> knee/1

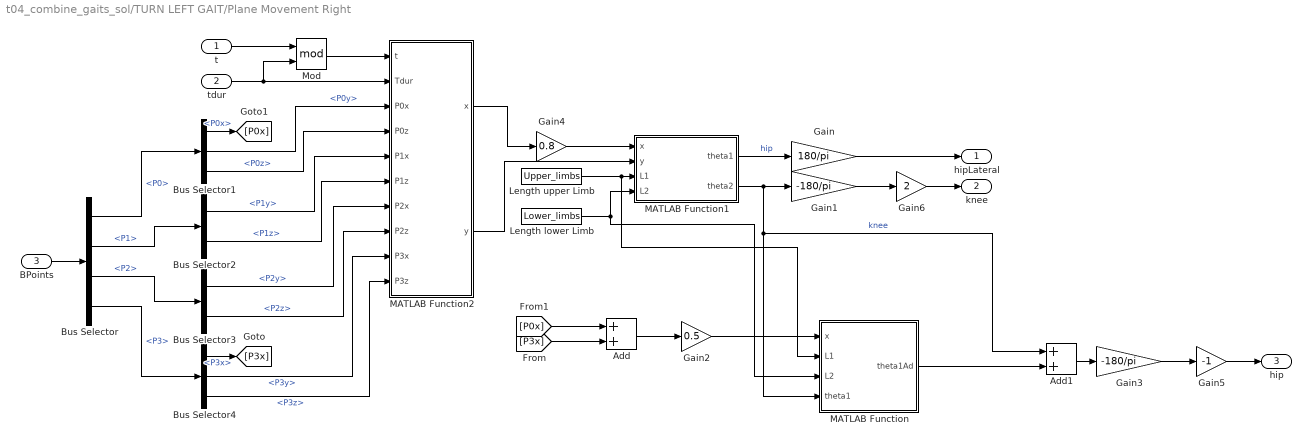
== system t04_combine_gaits_sol/TURN LEFT GAIT/Plane Movement Right ==
  t : Inport
  tdur : Inport  Port=2
  BPoints : Inport  Port=3
  Add : Sum
  Add1 : Sum
  Bus Selector : BusSelector  OutputSignals=P0,P1,P2,P3
  Bus Selector1 : BusSelector  OutputSignals=P0x,P0y,P0z
  Bus Selector2 : BusSelector  OutputSignals=P1y,P1z
  Bus Selector3 : BusSelector  OutputSignals=P2y,P2z
  Bus Selector4 : BusSelector  OutputSignals=P3x,P3y,P3z
  Gain : Gain  Gain=180/pi
  Gain1 : Gain  Gain=-180/pi
  Gain2 : Gain  Gain=0.5
  Gain3 : Gain  Gain=-180/pi
  Gain4 : Gain  Gain=0.8
  Gain5 : Gain  Gain=-1
  Gain6 : Gain  Gain=2
  Length lower Limb : Constant  Value=Lower_limbs
  Length upper Limb : Constant  Value=Upper_limbs
  MATLAB Function : MATLAB Function  TreatAsAtomicUnit=on
  MATLAB Function1 : MATLAB Function  TreatAsAtomicUnit=on
  MATLAB Function2 : MATLAB Function  TreatAsAtomicUnit=on
  Mod : Math  Operator=mod
  hipLateral : Outport
  knee : Outport  Port=2
  hip : Outport  Port=3
  wires:
  Gain4/1 -> MATLAB Function1/1(x)
  Gain3/1 -> Gain5/1
  Add1/1 -> Gain3/1
  Bus Selector1/1 -> [P0x]  "<P0x>"
  Bus Selector4/1 -> [P3x]  "<P3x>"
  MATLAB Function/1(theta1Ad) -> Add1/2
  [P3x] -> Add/2
  [P0x] -> Add/1
  Add/1 -> Gain2/1
  Gain2/1 -> MATLAB Function/1(x)
  Gain/1 -> hipLateral/1
  Gain1/1 -> Gain6/1
  Length lower Limb/1 -> MATLAB Function1/4(L2), MATLAB Function/3(L2)
  Length upper Limb/1 -> MATLAB Function1/3(L1), MATLAB Function/2(L1)
  t/1 -> Mod/1
  MATLAB Function1/1(theta1) -> Gain/1  "hip"
  tdur/1 -> MATLAB Function2/2(Tdur), Mod/2
  MATLAB Function1/2(theta2) -> Gain1/1, MATLAB Function/4(theta1), Add1/1  "knee"
  MATLAB Function2/1(x) -> Gain4/1
  MATLAB Function2/2(y) -> MATLAB Function1/2(y)
  Bus Selector/3 -> Bus Selector3/1  "<P2>"
  Bus Selector3/2 -> MATLAB Function2/8(P2z)  "<P2z>"
  Bus Selector2/1 -> MATLAB Function2/5(P1x)  "<P1y>"
  Bus Selector3/1 -> MATLAB Function2/7(P2x)  "<P2y>"
  Bus Selector4/2 -> MATLAB Function2/9(P3x)  "<P3y>"
  Bus Selector1/3 -> MATLAB Function2/4(P0z)  "<P0z>"
  Bus Selector/4 -> Bus Selector4/1  "<P3>"
  Bus Selector4/3 -> MATLAB Function2/10(P3z)  "<P3z>"
  Bus Selector/2 -> Bus Selector2/1  "<P1>"
  BPoints/1 -> Bus Selector/1
  Bus Selector1/2 -> MATLAB Function2/3(P0x)  "<P0y>"
  Bus Selector/1 -> Bus Selector1/1  "<P0>"
  Bus Selector2/2 -> MATLAB Function2/6(P1z)  "<P1z>"
  Mod/1 -> MATLAB Function2/1(t)
  Gain5/1 -> hip/1
  Gain6/1 -> knee/1

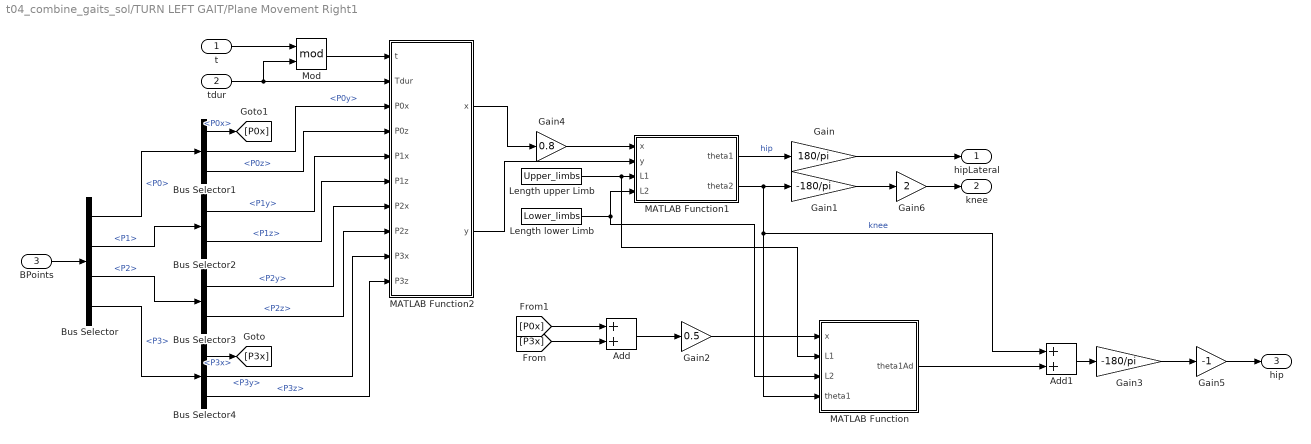
== system t04_combine_gaits_sol/TURN LEFT GAIT/Plane Movement Right1 ==
  t : Inport
  tdur : Inport  Port=2
  BPoints : Inport  Port=3
  Add : Sum
  Add1 : Sum
  Bus Selector : BusSelector  OutputSignals=P0,P1,P2,P3
  Bus Selector1 : BusSelector  OutputSignals=P0x,P0y,P0z
  Bus Selector2 : BusSelector  OutputSignals=P1y,P1z
  Bus Selector3 : BusSelector  OutputSignals=P2y,P2z
  Bus Selector4 : BusSelector  OutputSignals=P3x,P3y,P3z
  Gain : Gain  Gain=180/pi
  Gain1 : Gain  Gain=-180/pi
  Gain2 : Gain  Gain=0.5
  Gain3 : Gain  Gain=-180/pi
  Gain4 : Gain  Gain=0.8
  Gain5 : Gain  Gain=-1
  Gain6 : Gain  Gain=2
  Length lower Limb : Constant  Value=Lower_limbs
  Length upper Limb : Constant  Value=Upper_limbs
  MATLAB Function : MATLAB Function  TreatAsAtomicUnit=on
  MATLAB Function1 : MATLAB Function  TreatAsAtomicUnit=on
  MATLAB Function2 : MATLAB Function  TreatAsAtomicUnit=on
  Mod : Math  Operator=mod
  hipLateral : Outport
  knee : Outport  Port=2
  hip : Outport  Port=3
  wires:
  Gain6/1 -> knee/1
  Gain5/1 -> hip/1
  Mod/1 -> MATLAB Function2/1(t)
  Bus Selector2/2 -> MATLAB Function2/6(P1z)  "<P1z>"
  Bus Selector/1 -> Bus Selector1/1  "<P0>"
  Bus Selector1/2 -> MATLAB Function2/3(P0x)  "<P0y>"
  BPoints/1 -> Bus Selector/1
  Bus Selector/2 -> Bus Selector2/1  "<P1>"
  Bus Selector4/3 -> MATLAB Function2/10(P3z)  "<P3z>"
  Bus Selector/4 -> Bus Selector4/1  "<P3>"
  Bus Selector1/3 -> MATLAB Function2/4(P0z)  "<P0z>"
  Bus Selector4/2 -> MATLAB Function2/9(P3x)  "<P3y>"
  Bus Selector3/1 -> MATLAB Function2/7(P2x)  "<P2y>"
  Bus Selector2/1 -> MATLAB Function2/5(P1x)  "<P1y>"
  Bus Selector3/2 -> MATLAB Function2/8(P2z)  "<P2z>"
  Bus Selector/3 -> Bus Selector3/1  "<P2>"
  MATLAB Function2/2(y) -> MATLAB Function1/2(y)
  MATLAB Function2/1(x) -> Gain4/1
  MATLAB Function1/2(theta2) -> Add1/1, MATLAB Function/4(theta1), Gain1/1  "knee"
  tdur/1 -> Mod/2, MATLAB Function2/2(Tdur)
  MATLAB Function1/1(theta1) -> Gain/1  "hip"
  t/1 -> Mod/1
  Length upper Limb/1 -> MATLAB Function/2(L1), MATLAB Function1/3(L1)
  Length lower Limb/1 -> MATLAB Function/3(L2), MATLAB Function1/4(L2)
  Gain1/1 -> Gain6/1
  Gain/1 -> hipLateral/1
  Gain2/1 -> MATLAB Function/1(x)
  Add/1 -> Gain2/1
  [P0x] -> Add/1
  [P3x] -> Add/2
  MATLAB Function/1(theta1Ad) -> Add1/2
  Bus Selector4/1 -> [P3x]  "<P3x>"
  Bus Selector1/1 -> [P0x]  "<P0x>"
  Add1/1 -> Gain3/1
  Gain3/1 -> Gain5/1
  Gain4/1 -> MATLAB Function1/1(x)

== system t04_combine_gaits_sol/TURN LEFT GAIT/Subsystem ==
  t : Inport
  tdur : Inport  Port=2
  Add : Sum  Inputs=+-
  Add1 : Sum  Inputs=+-
  Add2 : Sum  Inputs=+-
  Gain : Gain  Gain=0.25
  Gain1 : Gain  Gain=0.5
  Gain2 : Gain  Gain=0.75
  t_0.25 : Outport
  t_0.5 : Outport  Port=2
  t_0.75 : Outport  Port=3
  wires:
  tdur/1 -> Gain/1, Gain2/1, Gain1/1
  Gain2/1 -> Add2/2
  Gain1/1 -> Add1/2
  t/1 -> Add/1, Add1/1, Add2/1
  Gain/1 -> Add/2
  Add/1 -> t_0.25/1
  Add1/1 -> t_0.5/1
  Add2/1 -> t_0.75/1

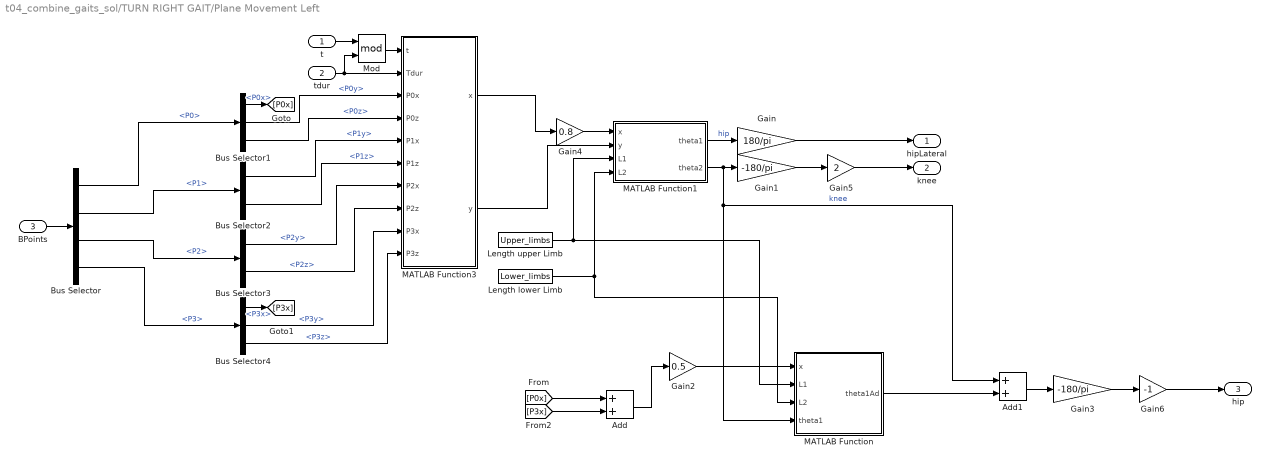
== system t04_combine_gaits_sol/TURN RIGHT GAIT/Plane Movement Left ==
  t : Inport
  tdur : Inport  Port=2
  BPoints : Inport  Port=3
  Add : Sum
  Add1 : Sum
  Bus Selector : BusSelector  OutputSignals=P0,P1,P2,P3
  Bus Selector1 : BusSelector  OutputSignals=P0x,P0y,P0z
  Bus Selector2 : BusSelector  OutputSignals=P1y,P1z
  Bus Selector3 : BusSelector  OutputSignals=P2y,P2z
  Bus Selector4 : BusSelector  OutputSignals=P3x,P3y,P3z
  Gain : Gain  Gain=180/pi
  Gain1 : Gain  Gain=-180/pi
  Gain2 : Gain  Gain=0.5
  Gain3 : Gain  Gain=-180/pi
  Gain4 : Gain  Gain=0.8
  Gain5 : Gain  Gain=2
  Gain6 : Gain  Gain=-1
  Length lower Limb : Constant  Value=Lower_limbs
  Length upper Limb : Constant  Value=Upper_limbs
  MATLAB Function : MATLAB Function  TreatAsAtomicUnit=on
  MATLAB Function1 : MATLAB Function  TreatAsAtomicUnit=on
  MATLAB Function3 : MATLAB Function  TreatAsAtomicUnit=on
  Mod : Math  Operator=mod
  hipLateral : Outport
  knee : Outport  Port=2
  hip : Outport  Port=3
  wires:
  Gain4/1 -> MATLAB Function1/1(x)
  Gain3/1 -> Gain6/1
  Add1/1 -> Gain3/1
  MATLAB Function/1(theta1Ad) -> Add1/2
  Bus Selector4/1 -> [P3x]  "<P3x>"
  Gain2/1 -> MATLAB Function/1(x)
  [P0x] -> Add/1
  [P3x] -> Add/2
  Add/1 -> Gain2/1
  Bus Selector1/1 -> [P0x]  "<P0x>"
  MATLAB Function3/2(y) -> MATLAB Function1/2(y)
  MATLAB Function3/1(x) -> Gain4/1
  MATLAB Function1/2(theta2) -> Gain1/1, MATLAB Function/4(theta1), Add1/1  "knee"
  tdur/1 -> Mod/2, MATLAB Function3/2(Tdur)
  MATLAB Function1/1(theta1) -> Gain/1  "hip"
  t/1 -> Mod/1
  Length upper Limb/1 -> MATLAB Function/2(L1), MATLAB Function1/3(L1)
  Length lower Limb/1 -> MATLAB Function/3(L2), MATLAB Function1/4(L2)
  Gain1/1 -> Gain5/1
  Gain/1 -> hipLateral/1
  Bus Selector/3 -> Bus Selector3/1  "<P2>"
  Bus Selector3/2 -> MATLAB Function3/8(P2z)  "<P2z>"
  Bus Selector2/1 -> MATLAB Function3/5(P1x)  "<P1y>"
  Bus Selector3/1 -> MATLAB Function3/7(P2x)  "<P2y>"
  Bus Selector4/2 -> MATLAB Function3/9(P3x)  "<P3y>"
  Bus Selector1/3 -> MATLAB Function3/4(P0z)  "<P0z>"
  Bus Selector/4 -> Bus Selector4/1  "<P3>"
  Bus Selector4/3 -> MATLAB Function3/10(P3z)  "<P3z>"
  Bus Selector/2 -> Bus Selector2/1  "<P1>"
  BPoints/1 -> Bus Selector/1
  Bus Selector1/2 -> MATLAB Function3/3(P0x)  "<P0y>"
  Bus Selector/1 -> Bus Selector1/1  "<P0>"
  Bus Selector2/2 -> MATLAB Function3/6(P1z)  "<P1z>"
  Mod/1 -> MATLAB Function3/1(t)
  Gain5/1 -> knee/1
  Gain6/1 -> hip/1

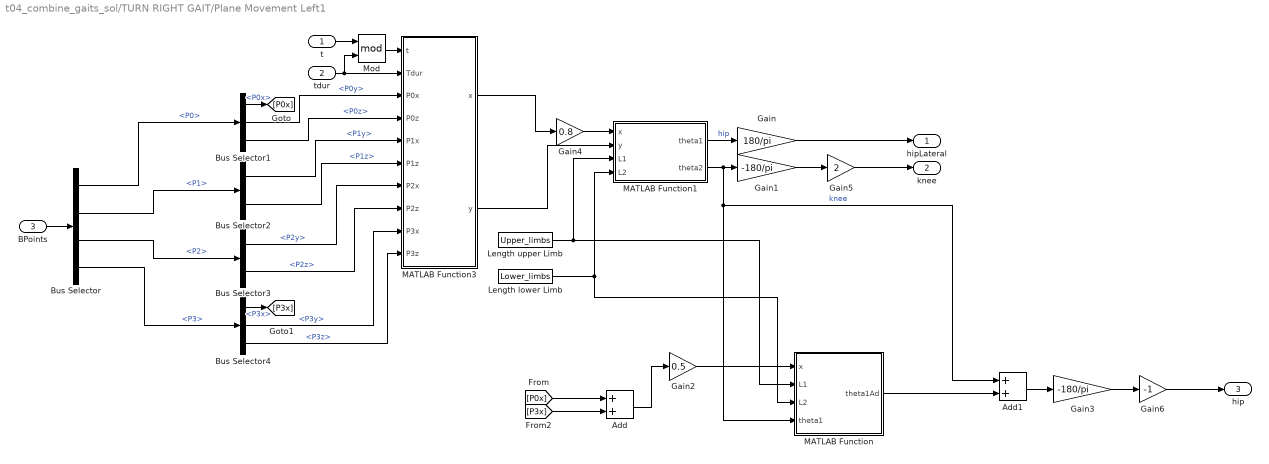
== system t04_combine_gaits_sol/TURN RIGHT GAIT/Plane Movement Left1 ==
  t : Inport
  tdur : Inport  Port=2
  BPoints : Inport  Port=3
  Add : Sum
  Add1 : Sum
  Bus Selector : BusSelector  OutputSignals=P0,P1,P2,P3
  Bus Selector1 : BusSelector  OutputSignals=P0x,P0y,P0z
  Bus Selector2 : BusSelector  OutputSignals=P1y,P1z
  Bus Selector3 : BusSelector  OutputSignals=P2y,P2z
  Bus Selector4 : BusSelector  OutputSignals=P3x,P3y,P3z
  Gain : Gain  Gain=180/pi
  Gain1 : Gain  Gain=-180/pi
  Gain2 : Gain  Gain=0.5
  Gain3 : Gain  Gain=-180/pi
  Gain4 : Gain  Gain=0.8
  Gain5 : Gain  Gain=2
  Gain6 : Gain  Gain=-1
  Length lower Limb : Constant  Value=Lower_limbs
  Length upper Limb : Constant  Value=Upper_limbs
  MATLAB Function : MATLAB Function  TreatAsAtomicUnit=on
  MATLAB Function1 : MATLAB Function  TreatAsAtomicUnit=on
  MATLAB Function3 : MATLAB Function  TreatAsAtomicUnit=on
  Mod : Math  Operator=mod
  hipLateral : Outport
  knee : Outport  Port=2
  hip : Outport  Port=3
  wires:
  Gain6/1 -> hip/1
  Gain5/1 -> knee/1
  Mod/1 -> MATLAB Function3/1(t)
  Bus Selector2/2 -> MATLAB Function3/6(P1z)  "<P1z>"
  Bus Selector/1 -> Bus Selector1/1  "<P0>"
  Bus Selector1/2 -> MATLAB Function3/3(P0x)  "<P0y>"
  BPoints/1 -> Bus Selector/1
  Bus Selector/2 -> Bus Selector2/1  "<P1>"
  Bus Selector4/3 -> MATLAB Function3/10(P3z)  "<P3z>"
  Bus Selector/4 -> Bus Selector4/1  "<P3>"
  Bus Selector1/3 -> MATLAB Function3/4(P0z)  "<P0z>"
  Bus Selector4/2 -> MATLAB Function3/9(P3x)  "<P3y>"
  Bus Selector3/1 -> MATLAB Function3/7(P2x)  "<P2y>"
  Bus Selector2/1 -> MATLAB Function3/5(P1x)  "<P1y>"
  Bus Selector3/2 -> MATLAB Function3/8(P2z)  "<P2z>"
  Bus Selector/3 -> Bus Selector3/1  "<P2>"
  Gain/1 -> hipLateral/1
  Gain1/1 -> Gain5/1
  Length lower Limb/1 -> MATLAB Function1/4(L2), MATLAB Function/3(L2)
  Length upper Limb/1 -> MATLAB Function1/3(L1), MATLAB Function/2(L1)
  t/1 -> Mod/1
  MATLAB Function1/1(theta1) -> Gain/1  "hip"
  tdur/1 -> MATLAB Function3/2(Tdur), Mod/2
  MATLAB Function1/2(theta2) -> Add1/1, MATLAB Function/4(theta1), Gain1/1  "knee"
  MATLAB Function3/1(x) -> Gain4/1
  MATLAB Function3/2(y) -> MATLAB Function1/2(y)
  Bus Selector1/1 -> [P0x]  "<P0x>"
  Add/1 -> Gain2/1
  [P3x] -> Add/2
  [P0x] -> Add/1
  Gain2/1 -> MATLAB Function/1(x)
  Bus Selector4/1 -> [P3x]  "<P3x>"
  MATLAB Function/1(theta1Ad) -> Add1/2
  Add1/1 -> Gain3/1
  Gain3/1 -> Gain6/1
  Gain4/1 -> MATLAB Function1/1(x)

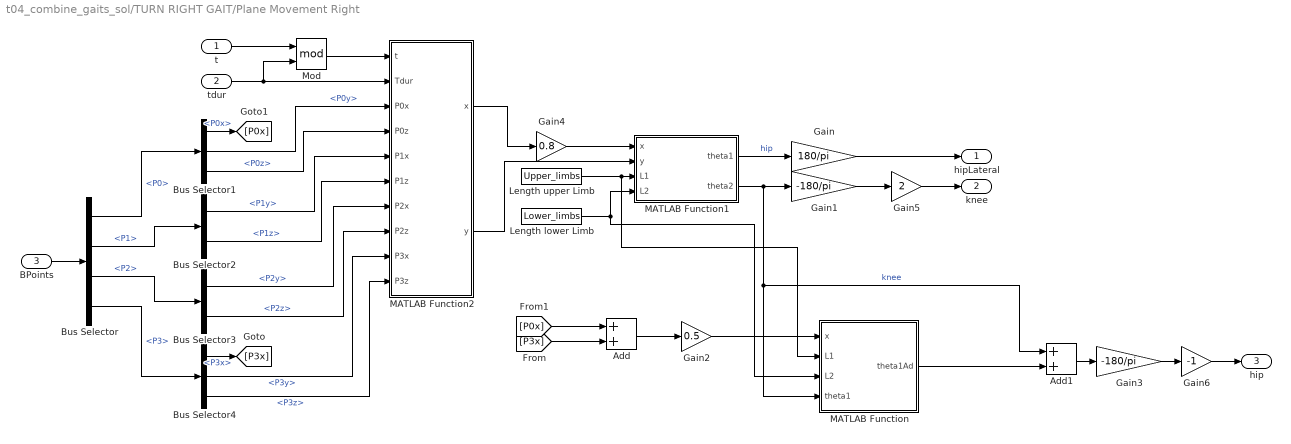
== system t04_combine_gaits_sol/TURN RIGHT GAIT/Plane Movement Right ==
  t : Inport
  tdur : Inport  Port=2
  BPoints : Inport  Port=3
  Add : Sum
  Add1 : Sum
  Bus Selector : BusSelector  OutputSignals=P0,P1,P2,P3
  Bus Selector1 : BusSelector  OutputSignals=P0x,P0y,P0z
  Bus Selector2 : BusSelector  OutputSignals=P1y,P1z
  Bus Selector3 : BusSelector  OutputSignals=P2y,P2z
  Bus Selector4 : BusSelector  OutputSignals=P3x,P3y,P3z
  Gain : Gain  Gain=180/pi
  Gain1 : Gain  Gain=-180/pi
  Gain2 : Gain  Gain=0.5
  Gain3 : Gain  Gain=-180/pi
  Gain4 : Gain  Gain=0.8
  Gain5 : Gain  Gain=2
  Gain6 : Gain  Gain=-1
  Length lower Limb : Constant  Value=Lower_limbs
  Length upper Limb : Constant  Value=Upper_limbs
  MATLAB Function : MATLAB Function  TreatAsAtomicUnit=on
  MATLAB Function1 : MATLAB Function  TreatAsAtomicUnit=on
  MATLAB Function2 : MATLAB Function  TreatAsAtomicUnit=on
  Mod : Math  Operator=mod
  hipLateral : Outport
  knee : Outport  Port=2
  hip : Outport  Port=3
  wires:
  Gain4/1 -> MATLAB Function1/1(x)
  Gain3/1 -> Gain6/1
  Add1/1 -> Gain3/1
  Bus Selector1/1 -> [P0x]  "<P0x>"
  Bus Selector4/1 -> [P3x]  "<P3x>"
  MATLAB Function/1(theta1Ad) -> Add1/2
  [P3x] -> Add/2
  [P0x] -> Add/1
  Add/1 -> Gain2/1
  Gain2/1 -> MATLAB Function/1(x)
  Gain/1 -> hipLateral/1
  Gain1/1 -> Gain5/1
  Length lower Limb/1 -> MATLAB Function1/4(L2), MATLAB Function/3(L2)
  Length upper Limb/1 -> MATLAB Function1/3(L1), MATLAB Function/2(L1)
  t/1 -> Mod/1
  MATLAB Function1/1(theta1) -> Gain/1  "hip"
  tdur/1 -> MATLAB Function2/2(Tdur), Mod/2
  MATLAB Function1/2(theta2) -> Gain1/1, MATLAB Function/4(theta1), Add1/1  "knee"
  MATLAB Function2/1(x) -> Gain4/1
  MATLAB Function2/2(y) -> MATLAB Function1/2(y)
  Bus Selector/3 -> Bus Selector3/1  "<P2>"
  Bus Selector3/2 -> MATLAB Function2/8(P2z)  "<P2z>"
  Bus Selector2/1 -> MATLAB Function2/5(P1x)  "<P1y>"
  Bus Selector3/1 -> MATLAB Function2/7(P2x)  "<P2y>"
  Bus Selector4/2 -> MATLAB Function2/9(P3x)  "<P3y>"
  Bus Selector1/3 -> MATLAB Function2/4(P0z)  "<P0z>"
  Bus Selector/4 -> Bus Selector4/1  "<P3>"
  Bus Selector4/3 -> MATLAB Function2/10(P3z)  "<P3z>"
  Bus Selector/2 -> Bus Selector2/1  "<P1>"
  BPoints/1 -> Bus Selector/1
  Bus Selector1/2 -> MATLAB Function2/3(P0x)  "<P0y>"
  Bus Selector/1 -> Bus Selector1/1  "<P0>"
  Bus Selector2/2 -> MATLAB Function2/6(P1z)  "<P1z>"
  Mod/1 -> MATLAB Function2/1(t)
  Gain5/1 -> knee/1
  Gain6/1 -> hip/1

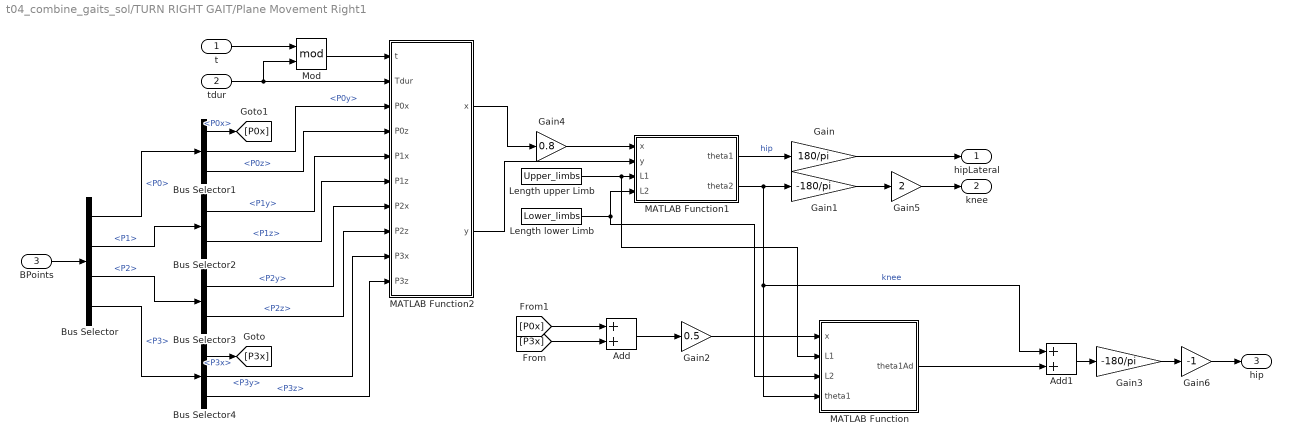
== system t04_combine_gaits_sol/TURN RIGHT GAIT/Plane Movement Right1 ==
  t : Inport
  tdur : Inport  Port=2
  BPoints : Inport  Port=3
  Add : Sum
  Add1 : Sum
  Bus Selector : BusSelector  OutputSignals=P0,P1,P2,P3
  Bus Selector1 : BusSelector  OutputSignals=P0x,P0y,P0z
  Bus Selector2 : BusSelector  OutputSignals=P1y,P1z
  Bus Selector3 : BusSelector  OutputSignals=P2y,P2z
  Bus Selector4 : BusSelector  OutputSignals=P3x,P3y,P3z
  Gain : Gain  Gain=180/pi
  Gain1 : Gain  Gain=-180/pi
  Gain2 : Gain  Gain=0.5
  Gain3 : Gain  Gain=-180/pi
  Gain4 : Gain  Gain=0.8
  Gain5 : Gain  Gain=2
  Gain6 : Gain  Gain=-1
  Length lower Limb : Constant  Value=Lower_limbs
  Length upper Limb : Constant  Value=Upper_limbs
  MATLAB Function : MATLAB Function  TreatAsAtomicUnit=on
  MATLAB Function1 : MATLAB Function  TreatAsAtomicUnit=on
  MATLAB Function2 : MATLAB Function  TreatAsAtomicUnit=on
  Mod : Math  Operator=mod
  hipLateral : Outport
  knee : Outport  Port=2
  hip : Outport  Port=3
  wires:
  Gain6/1 -> hip/1
  Gain5/1 -> knee/1
  Mod/1 -> MATLAB Function2/1(t)
  Bus Selector2/2 -> MATLAB Function2/6(P1z)  "<P1z>"
  Bus Selector/1 -> Bus Selector1/1  "<P0>"
  Bus Selector1/2 -> MATLAB Function2/3(P0x)  "<P0y>"
  BPoints/1 -> Bus Selector/1
  Bus Selector/2 -> Bus Selector2/1  "<P1>"
  Bus Selector4/3 -> MATLAB Function2/10(P3z)  "<P3z>"
  Bus Selector/4 -> Bus Selector4/1  "<P3>"
  Bus Selector1/3 -> MATLAB Function2/4(P0z)  "<P0z>"
  Bus Selector4/2 -> MATLAB Function2/9(P3x)  "<P3y>"
  Bus Selector3/1 -> MATLAB Function2/7(P2x)  "<P2y>"
  Bus Selector2/1 -> MATLAB Function2/5(P1x)  "<P1y>"
  Bus Selector3/2 -> MATLAB Function2/8(P2z)  "<P2z>"
  Bus Selector/3 -> Bus Selector3/1  "<P2>"
  MATLAB Function2/2(y) -> MATLAB Function1/2(y)
  MATLAB Function2/1(x) -> Gain4/1
  MATLAB Function1/2(theta2) -> Add1/1, MATLAB Function/4(theta1), Gain1/1  "knee"
  tdur/1 -> Mod/2, MATLAB Function2/2(Tdur)
  MATLAB Function1/1(theta1) -> Gain/1  "hip"
  t/1 -> Mod/1
  Length upper Limb/1 -> MATLAB Function/2(L1), MATLAB Function1/3(L1)
  Length lower Limb/1 -> MATLAB Function/3(L2), MATLAB Function1/4(L2)
  Gain1/1 -> Gain5/1
  Gain/1 -> hipLateral/1
  Gain2/1 -> MATLAB Function/1(x)
  Add/1 -> Gain2/1
  [P0x] -> Add/1
  [P3x] -> Add/2
  MATLAB Function/1(theta1Ad) -> Add1/2
  Bus Selector4/1 -> [P3x]  "<P3x>"
  Bus Selector1/1 -> [P0x]  "<P0x>"
  Add1/1 -> Gain3/1
  Gain3/1 -> Gain6/1
  Gain4/1 -> MATLAB Function1/1(x)

== system t04_combine_gaits_sol/TURN RIGHT GAIT/Subsystem ==
  t : Inport
  tdur : Inport  Port=2
  Add : Sum  Inputs=+-
  Add1 : Sum  Inputs=+-
  Add2 : Sum  Inputs=+-
  Gain : Gain  Gain=0.25
  Gain1 : Gain  Gain=0.5
  Gain2 : Gain  Gain=0.75
  t_0.25 : Outport
  t_0.5 : Outport  Port=2
  t_0.75 : Outport  Port=3
  wires:
  tdur/1 -> Gain/1, Gain2/1, Gain1/1
  Gain2/1 -> Add2/2
  Gain1/1 -> Add1/2
  t/1 -> Add/1, Add1/1, Add2/1
  Gain/1 -> Add/2
  Add/1 -> t_0.25/1
  Add1/1 -> t_0.5/1
  Add2/1 -> t_0.75/1
